simulink model "controllo_robusto"  (R2022b)
settings: Solver=VariableStepAuto  StartTime=0.0  StopTime=40  RelTol=1e-3
values from neighbouring files (symbols this model uses):
  D = [zeros(4); eye(4)]    [controllo_script.m]
  Kd_cr = 200*eye(4)    [controllo_script.m]
  Kp_cr = (Kd_cr^2)/2 * eye(4)    [controllo_script.m]
  Q = lyap(Htilde, P)    [controllo_script.m]
  T = T_A * T_B    [DH_dinamica.m]    (also in traiettoria_script.m = 0.001)
  theta1_0 = pi/2 - angolo    [CLIK_script.m]
  theta2_0 = 2*angolo    [CLIK_script.m]
undefined symbols (not defined in the file or in its folder): DiscIntNeverNeededParam
settings Model: Creator=Principale  LastModifiedBy=Michele
settings DataIOCC: ReturnWorkspaceOutputs=off

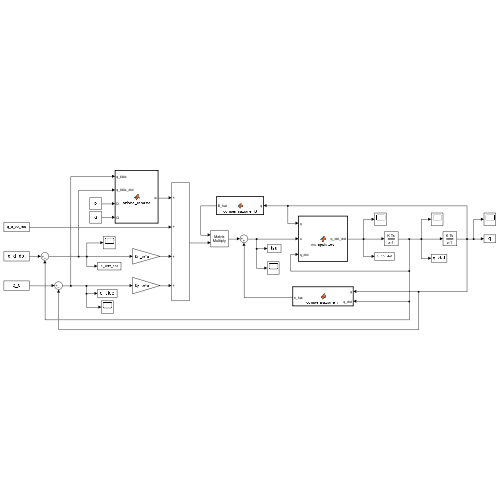
[thumbnail: Simulink's stored preview of the top-level diagram]
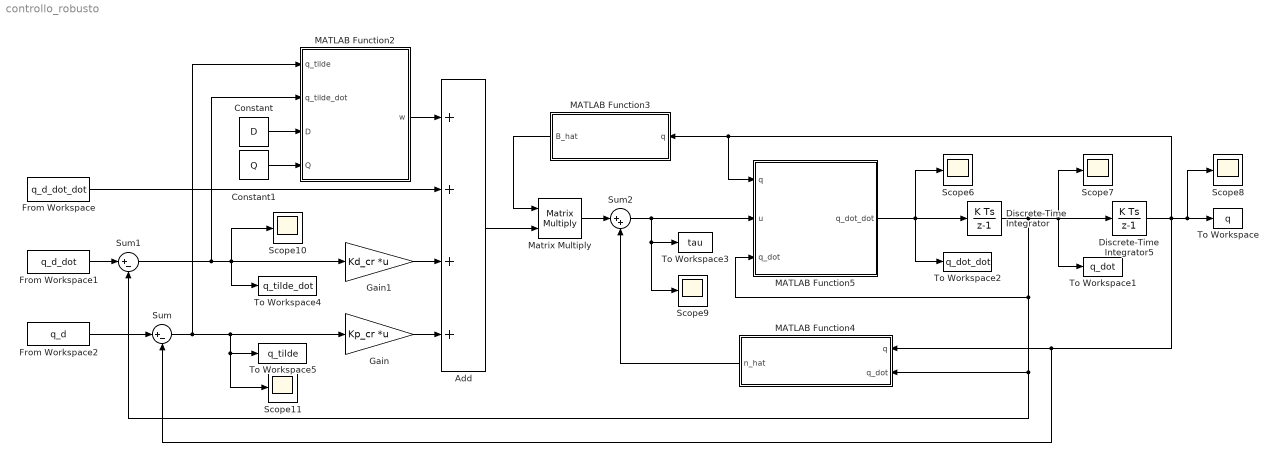
== system controllo_robusto ==
  Add : Sum  Inputs=++++
  Constant : Constant  Value=D  VectorParams1D=off
  Constant1 : Constant  Value=Q  VectorParams1D=off
  Discrete-Time Integrator : DiscreteIntegrator  InitialCondition=[0 0 0 0]'  SampleTime=-1  ICPrevOutput=DiscIntNeverNeededParam  ICPrevScaledInput=DiscIntNeverNeededParam
  Discrete-Time Integrator5 : DiscreteIntegrator  InitialCondition=[theta1_0 theta2_0 -0.25 0]'  SampleTime=-1  ICPrevOutput=DiscIntNeverNeededParam  ICPrevScaledInput=DiscIntNeverNeededParam
  From Workspace : FromWorkspace  VariableName=q_d_dot_dot  SampleTime=T
  From Workspace1 : FromWorkspace  VariableName=q_d_dot  SampleTime=T
  From Workspace2 : FromWorkspace  VariableName=q_d  SampleTime=T
  Gain : Gain  Gain=Kp_cr  Multiplication=Matrix(K*u)
  Gain1 : Gain  Gain=Kd_cr  Multiplication=Matrix(K*u)
  MATLAB Function2 : MATLAB Function  TreatAsAtomicUnit=on
  MATLAB Function3 : MATLAB Function  TreatAsAtomicUnit=on
  MATLAB Function4 : MATLAB Function  TreatAsAtomicUnit=on
  MATLAB Function5 : MATLAB Function  TreatAsAtomicUnit=on
  Matrix Multiply : Product  Multiplication=Matrix(*)
  Scope{6..11} (6 alike) : Scope
  Sum : Sum  Inputs=|+-
  Sum1 : Sum  Inputs=|+-
  Sum2 : Sum  Inputs=|++
  To Workspace : ToWorkspace  VariableName=q  SaveFormat=Structure With Time  SampleTime=-1
  To Workspace1 : ToWorkspace  VariableName=q_dot  SaveFormat=Structure With Time  SampleTime=-1
  To Workspace2 : ToWorkspace  VariableName=q_dot_dot  SaveFormat=Structure With Time  SampleTime=-1
  To Workspace3 : ToWorkspace  VariableName=tau  SaveFormat=Structure With Time  SampleTime=-1
  To Workspace4 : ToWorkspace  VariableName=q_tilde_dot  SaveFormat=Structure With Time  SampleTime=-1
  To Workspace5 : ToWorkspace  VariableName=q_tilde  SaveFormat=Structure With Time  SampleTime=-1
  wires:
  Sum/1 -> MATLAB Function2/1(q_tilde), To Workspace5/1, Scope11/1, Gain/1
  From Workspace2/1 -> Sum/1
  From Workspace1/1 -> Sum1/1
  Sum1/1 -> MATLAB Function2/2(q_tilde_dot), To Workspace4/1, Scope10/1, Gain1/1
  Gain1/1 -> Add/3
  Gain/1 -> Add/4
  MATLAB Function4/1(n_hat) -> Sum2/2
  MATLAB Function5/1(q_dot_dot) -> Discrete-Time Integrator/1, To Workspace2/1, Scope6/1
  Discrete-Time Integrator/1 -> Discrete-Time Integrator5/1, To Workspace1/1, Scope7/1, Sum1/2, MATLAB Function4/2(q_dot), MATLAB Function5/3(q_dot)
  Discrete-Time Integrator5/1 -> To Workspace/1, Scope8/1, Sum/2, MATLAB Function4/1(q), MATLAB Function5/1(q), MATLAB Function3/1(q)
  Sum2/1 -> MATLAB Function5/2(u), Scope9/1, To Workspace3/1
  Constant/1 -> MATLAB Function2/3(D)
  Constant1/1 -> MATLAB Function2/4(Q)
  From Workspace/1 -> Add/2
  MATLAB Function2/1(w) -> Add/1
  MATLAB Function3/1(B_hat) -> Matrix Multiply/1
  Add/1 -> Matrix Multiply/2
  Matrix Multiply/1 -> Sum2/1

== matlab function controllo_robusto/MATLAB Function3 ==
  data: q input; B_hat output
function B_hat = compensazione_B(q)

    q1 = q(1);
    q2 = q(2);
    
    B = [10*(cos(q1)/2 + (cos(q1)*cos(q2))/2 - (sin(q1)*sin(q2))/2)^2 + 20*(cos(q1)/2 + (cos(q1)*cos(q2))/4 - (sin(q1)*sin(q2))/4)^2 + 10*(sin(q1)/2 + (cos(q1)*sin(q2))/2 + (cos(q2)*sin(q1))/2)^2 + 20*(sin(q1)/2 + (cos(q1)*sin(q2))/4 + (cos(q2)*sin(q1))/4)^2 + (5*cos(q1)^2)/4 + (5*sin(q1)^2)/4 + 4513/500, 10*((cos(q1)*cos(q2))/2 - (sin(q1)*sin(q2))/2)*(cos(q1)/2 + (cos(q1)*cos(q2))/2 - (sin(q1)*sin(q2))/2) + 20*((cos(q1)*cos(q2))/4 - (sin(q1)*sin(q2))/4)*(cos(q1)/2 + (cos(q1)*cos(q2))/4 - (sin(q1)*sin(q2))/4) + 10*((cos(q1)*sin(q2))/2 + (cos(q2)*sin(q1))/2)*(sin(q1)/2 + (cos(q1)*sin(q2))/2 + (cos(q2)*sin(q1))/2) + 20*((cos(q1)*sin(q2))/4 + (cos(q2)*sin(q1))/4)*(sin(q1)/2 + (cos(q1)*sin(q2))/4 + (cos(q2)*sin(q1))/4) + 627/125, 1/3, -51/50;
    10*((cos(q1)*cos(q2))/2 - (sin(q1)*sin(q2))/2)*(cos(q1)/2 + (cos(q1)*cos(q2))/2 - (sin(q1)*sin(q2))/2) + 20*((cos(q1)*cos(q2))/4 - (sin(q1)*sin(q2))/4)*(cos(q1)/2 + (cos(q1)*cos(q2))/4 - (sin(q1)*sin(q2))/4) + 10*((cos(q1)*sin(q2))/2 + (cos(q2)*sin(q1))/2)*(sin(q1)/2 + (cos(q1)*sin(q2))/2 + (cos(q2)*sin(q1))/2) + 20*((cos(q1)*sin(q2))/4 + (cos(q2)*sin(q1))/4)*(sin(q1)/2 + (cos(q1)*sin(q2))/4 + (cos(q2)*sin(q1))/4) + 627/125, 10*((cos(q1)*cos(q2))/2 - (sin(q1)*sin(q2))/2)^2 + 10*((cos(q1)*sin(q2))/2 + (cos(q2)*sin(q1))/2)^2 + 20*((cos(q1)*cos(q2))/4 - (sin(q1)*sin(q2))/4)^2 + 20*((cos(q1)*sin(q2))/4 + (cos(q2)*sin(q1))/4)^2 + 627/125, 1/4, -51/50;
    1/4, 1/4, 45/2, 0;
    -51/50, -51/50, 0, 7/5];
    
    % Costruisco B_hat estraendo solo i termini sulla diagonale di B
    B_hat = diag(diag(B));   
end

== matlab function controllo_robusto/MATLAB Function2 ==
  data: q_tilde input; w output; q_tilde_dot input; D input; Q input
function w  = azione_robusta(q_tilde, q_tilde_dot, D, Q)

    xi = [q_tilde; q_tilde_dot];

    z = D'*Q*xi;

    ro = 1;
    epsilon = 0.1;

    if(norm(z)>=epsilon)
        w = ro*z/norm(z);
    else 
        w = ro*z/epsilon;     
    end
end

== matlab function controllo_robusto/MATLAB Function4 ==
  data: q input; n_hat output; q_dot input
function n_hat = compensazione_n(q,q_dot)

    % n_hat compensa solo la coppia di gravità
    n_hat=[0;0;98.1;0];
end

== matlab function controllo_robusto/MATLAB Function5 ==
  data: q input; q_dot_dot output; u input; q_dot input
function q_dot_dot = manipolatore(q, u, q_dot)

    q1 = q(1);
    q2 = q(2);
    q3 = q(3);
    q4 = q(4);
    
    q_dot1 = q_dot(1);
    q_dot2 = q_dot(2);
    q_dot3 = q_dot(3);
    q_dot4 = q_dot(4);
    
    B = [14*(cos(q1)/2 + (cos(q1)*cos(q2))/2 - (sin(q1)*sin(q2))/2)^2 + 20*(cos(q1)/2 + (cos(q1)*cos(q2))/4 - (sin(q1)*sin(q2))/4)^2 + 14*(sin(q1)/2 + (cos(q1)*sin(q2))/2 + (cos(q2)*sin(q1))/2)^2 + 20*(sin(q1)/2 + (cos(q1)*sin(q2))/4 + (cos(q2)*sin(q1))/4)^2 + (5*cos(q1)^2)/4 + (5*sin(q1)^2)/4 + 4513/500, 14*((cos(q1)*cos(q2))/2 - (sin(q1)*sin(q2))/2)*(cos(q1)/2 + (cos(q1)*cos(q2))/2 - (sin(q1)*sin(q2))/2) + 20*((cos(q1)*cos(q2))/4 - (sin(q1)*sin(q2))/4)*(cos(q1)/2 + (cos(q1)*cos(q2))/4 - (sin(q1)*sin(q2))/4) + 14*((cos(q1)*sin(q2))/2 + (cos(q2)*sin(q1))/2)*(sin(q1)/2 + (cos(q1)*sin(q2))/2 + (cos(q2)*sin(q1))/2) + 20*((cos(q1)*sin(q2))/4 + (cos(q2)*sin(q1))/4)*(sin(q1)/2 + (cos(q1)*sin(q2))/4 + (cos(q2)*sin(q1))/4) + 627/125,  1/4, -51/50;
    14*((cos(q1)*cos(q2))/2 - (sin(q1)*sin(q2))/2)*(cos(q1)/2 + (cos(q1)*cos(q2))/2 - (sin(q1)*sin(q2))/2) + 20*((cos(q1)*cos(q2))/4 - (sin(q1)*sin(q2))/4)*(cos(q1)/2 + (cos(q1)*cos(q2))/4 - (sin(q1)*sin(q2))/4) + 14*((cos(q1)*sin(q2))/2 + (cos(q2)*sin(q1))/2)*(sin(q1)/2 + (cos(q1)*sin(q2))/2 + (cos(q2)*sin(q1))/2) + 20*((cos(q1)*sin(q2))/4 + (cos(q2)*sin(q1))/4)*(sin(q1)/2 + (cos(q1)*sin(q2))/4 + (cos(q2)*sin(q1))/4) + 627/125,                                                                                                                                                                                                                         14*((cos(q1)*cos(q2))/2 - (sin(q1)*sin(q2))/2)^2 + 14*((cos(q1)*sin(q2))/2 + (cos(q2)*sin(q1))/2)^2 + 20*((cos(q1)*cos(q2))/4 - (sin(q1)*sin(q2))/4)^2 + 20*((cos(q1)*sin(q2))/4 + (cos(q2)*sin(q1))/4)^2 + 627/125,  1/4, -51/50;
                                                                                                                                                                                                                                                                                                                                                                                                                                           1/4,                                                                                                                                                                                                                                                                                                                                                                                                                                         1/4, 53/2,      0;
                                                                                                                                                                                                                                                                                                                                                                                                                                        -51/50,                                                                                                                                                                                                                                                                                                                                                                                                                                      -51/50,    0,    7/5];
    
    n = [q_dot2/20000 + (q_dot1*(q_dot2*(14*((cos(q1)*sin(q2))/2 + (cos(q2)*sin(q1))/2)*(cos(q1)/2 + (cos(q1)*cos(q2))/2 - (sin(q1)*sin(q2))/2) + 20*((cos(q1)*sin(q2))/4 + (cos(q2)*sin(q1))/4)*(cos(q1)/2 + (cos(q1)*cos(q2))/4 - (sin(q1)*sin(q2))/4) - 14*((cos(q1)*cos(q2))/2 - (sin(q1)*sin(q2))/2)*(sin(q1)/2 + (cos(q1)*sin(q2))/2 + (cos(q2)*sin(q1))/2) - 20*((cos(q1)*cos(q2))/4 - (sin(q1)*sin(q2))/4)*(sin(q1)/2 + (cos(q1)*sin(q2))/4 + (cos(q2)*sin(q1))/4)) + q_dot1*(28*((cos(q1)*sin(q2))/2 + (cos(q2)*sin(q1))/2)*(cos(q1)/2 + (cos(q1)*cos(q2))/2 - (sin(q1)*sin(q2))/2) + 40*((cos(q1)*sin(q2))/4 + (cos(q2)*sin(q1))/4)*(cos(q1)/2 + (cos(q1)*cos(q2))/4 - (sin(q1)*sin(q2))/4) - 28*((cos(q1)*cos(q2))/2 - (sin(q1)*sin(q2))/2)*(sin(q1)/2 + (cos(q1)*sin(q2))/2 + (cos(q2)*sin(q1))/2) - 40*((cos(q1)*cos(q2))/4 - (sin(q1)*sin(q2))/4)*(sin(q1)/2 + (cos(q1)*sin(q2))/4 + (cos(q2)*sin(q1))/4))))/2 - (q_dot1*q_dot2*(14*((cos(q1)*sin(q2))/2 + (cos(q2)*sin(q1))/2)*(cos(q1)/2 + (cos(q1)*cos(q2))/2 - (sin(q1)*sin(q2))/2) + 20*((cos(q1)*sin(q2))/4 + (cos(q2)*sin(q1))/4)*(cos(q1)/2 + (cos(q1)*cos(q2))/4 - (sin(q1)*sin(q2))/4) - 14*((cos(q1)*cos(q2))/2 - (sin(q1)*sin(q2))/2)*(sin(q1)/2 + (cos(q1)*sin(q2))/2 + (cos(q2)*sin(q1))/2) - 20*((cos(q1)*cos(q2))/4 - (sin(q1)*sin(q2))/4)*(sin(q1)/2 + (cos(q1)*sin(q2))/4 + (cos(q2)*sin(q1))/4)))/2];
    
    q_dot_dot = B\(u-n);
end
